simulink model "pattern_separation"  (R2019b)
settings: Solver=FixedStepAuto  StartTime=1  StopTime=simulationtime  FixedStep=stepsize  RelTol=1e-3
values from neighbouring files (symbols this model uses):
  a1 = 0.02    [simulation.m]
  a2 = 0.02    [simulation.m]
  b1 = 0.025    [simulation.m]
  b2 = 0.04    [simulation.m]
  c1 = -65    [simulation.m]
  C1 = normrnd(100,10,[1,nrofgranulecells])    [simulation.m]
  c2 = -65    [simulation.m]
  C2 = normrnd(100,10,[1,nrofinterneurons])    [simulation.m]
  d1 = 6    [simulation.m]
  d2 = 2    [simulation.m]
  inputset = inputsets{no_input}    [simulation.m]
  k1 = 0.25    [simulation.m]
  k2 = 0.25    [simulation.m]
  minimum_saturation_limit_1 = -80    [simulation.m]
  minimum_saturation_limit_2 = -100    [simulation.m]
  noumberofevents = 500    [simulation.m]
  Re = 230    [simulation.m]
  simulationtime = 2000    [simulation.m]
  stepsize = 1    [simulation.m]
  ve1 = -5    [simulation.m]
  ve2 = -80    [simulation.m]
  vr1 = -60    [simulation.m]
  vr2 = -65    [simulation.m]
  vt1 = -55    [simulation.m]
  vt2 = -48    [simulation.m]
undefined symbols (not defined in the file or in its folder): conductancemaxima1, conductancemaxima2, conductancemaxima3, decaytimes1, decaytimes2, decaytimes3, DiscIntNeverNeededParam, Nd, trace
(part 3 of 5)

== system pattern_separation/PV+ interneuron 2/interneuron ==
  postsynaptic current : Inport
  AHP or ADP : Constant  Value=c2  SampleTime=-1
  AP threshold potential : Constant  Value=vt2  SampleTime=-1
  Add : Sum  Inputs=+-
  Add2 : Sum  Inputs=+-
  Add3 : Sum  Inputs=+-
  Constant1 : Constant  Value=d2  SampleTime=-1
  Gain1 : Gain  Gain=b2
  Gain2 : Gain  Gain=k2
  Integrator : Integrator  ExternalReset=rising  InitialCondition=d2
  Integrator1 : Integrator  ExternalReset=rising  InitialCondition=vr2  LimitOutput=on  UpperSaturationLimit=30  LowerSaturationLimit=minimum_saturation_limit_2
  Memory : Memory  InheritSampleTime=on
  Memory1 : Memory  InitialCondition=vr2  InheritSampleTime=on
  Product : Product
  f' : Sum  Inputs=++-
  f'' : Sum  Inputs=+-
  membrne capacitance : Gain  Gain=1/C2(2)
  reset function : MATLAB Function  TreatAsAtomicUnit=on
  resting membrane potential : Constant  Value=vr2  SampleTime=-1
  time constant of relative refractory period : Gain  Gain=a2
  output : Outport
  wires:
  time constant of relative refractory period/1 -> Integrator/1  "u"
  Constant1/1 -> reset function/3(d)
  f''/1 -> time constant of relative refractory period/1
  membrne capacitance/1 -> Integrator1/1  "v"
  resting membrane potential/1 -> Add2/2, Add/2
  AHP or ADP/1 -> reset function/2(c)
  Add2/1 -> Product/1
  reset function/3(r) -> output/1, Integrator1/2, Integrator/2
  Gain1/1 -> f''/1
  Add3/1 -> Product/2
  Memory1/1 -> reset function/1(v)
  reset function/1(v1) -> Add/1, Add2/1, Add3/1
  reset function/2(u1) -> f''/2, f'/3
  Memory/1 -> reset function/4(u)
  Add/1 -> Gain1/1
  Integrator/1 -> Memory/1  "u"
  AP threshold potential/1 -> Add3/2
  Integrator1/1 -> Memory1/1  "v"
  f'/1 -> membrne capacitance/1
  Product/1 -> Gain2/1
  Gain2/1 -> f'/2
  postsynaptic current/1 -> f'/1

== system pattern_separation/PV+ interneuron 2/single exp EPSCs generator (ff synapse) ==
  event time : Inport
  decay time constant : Inport  Port=2
  conductance maximum : Inport  Port=3
  Add1 : Sum  Inputs=+-
  MATLAB Function : MATLAB Function  TreatAsAtomicUnit=on
  Multiply : Gain  Gain=-1
  Product : Product
  Product1 : Product  Inputs=*/
  Product2 : Product
  current reversal potential : Constant  Value=ve1  SampleTime=-1
  resting membrane potential : Constant  Value=vr1  SampleTime=-1
  postsynaptic current : Outport
  wires:
  decay time constant/1 -> Product1/2
  Product/1 -> postsynaptic current/1  "postsynaptic current"
  resting membrane potential/1 -> Add1/1
  current reversal potential/1 -> Add1/2
  conductance maximum/1 -> Product2/2
  Product2/1 -> Product/2  "conductance"
  Add1/1 -> Multiply/1
  Product1/1 -> MATLAB Function/1(inp)
  MATLAB Function/1(exponential) -> Product2/1
  event time/1 -> Product1/1
  Multiply/1 -> Product/1

== system pattern_separation/granule cell 1/granule cell ==
  postsynaptic current : Inport
  AHP or ADP : Constant  Value=c1  SampleTime=-1
  AP threshold potential : Constant  Value=vt1  SampleTime=-1
  Add : Sum  Inputs=+-
  Add2 : Sum  Inputs=+-
  Add3 : Sum  Inputs=+-
  Constant1 : Constant  Value=d1  SampleTime=-1
  Gain1 : Gain  Gain=b1
  Gain2 : Gain  Gain=k1
  Integrator : Integrator  ExternalReset=rising  InitialCondition=d1
  Integrator1 : Integrator  ExternalReset=rising  InitialCondition=vr1  LimitOutput=on  UpperSaturationLimit=30  LowerSaturationLimit=minimum_saturation_limit_1
  Memory : Memory  InheritSampleTime=on
  Memory1 : Memory  InitialCondition=vr1  InheritSampleTime=on
  Product : Product
  f' : Sum  Inputs=++-
  f'' : Sum  Inputs=+-
  membrne capacitance : Gain  Gain=1/C1(1)
  reset function : MATLAB Function  TreatAsAtomicUnit=on
  resting membrane potential : Constant  Value=vr1  SampleTime=-1
  time constant of relative refractory period : Gain  Gain=a1
  v : Outport
  output : Outport  Port=2
  wires:
  time constant of relative refractory period/1 -> Integrator/1  "u"
  Constant1/1 -> reset function/3(d)
  f''/1 -> time constant of relative refractory period/1
  membrne capacitance/1 -> Integrator1/1  "v"
  resting membrane potential/1 -> Add2/2, Add/2
  AHP or ADP/1 -> reset function/2(c)
  Add2/1 -> Product/1
  reset function/3(r) -> output/1, Integrator1/2, Integrator/2
  Gain1/1 -> f''/1
  Add3/1 -> Product/2
  Memory1/1 -> reset function/1(v)
  reset function/1(v1) -> Add/1, Add2/1, Add3/1
  reset function/2(u1) -> f''/2, f'/3
  Memory/1 -> reset function/4(u)
  Add/1 -> Gain1/1
  Integrator/1 -> Memory/1  "u"
  AP threshold potential/1 -> Add3/2
  Integrator1/1 -> v/1, Memory1/1  "v"
  f'/1 -> membrne capacitance/1
  Product/1 -> Gain2/1
  Gain2/1 -> f'/2
  postsynaptic current/1 -> f'/1

== system pattern_separation/granule cell 1/single exp EPSCs generator (recurrent synapse) ==
  event time : Inport
  decay time constant : Inport  Port=2
  conductance maximum : Inport  Port=3
  Add1 : Sum  Inputs=+-
  MATLAB Function : MATLAB Function  TreatAsAtomicUnit=on
  Multiply : Gain  Gain=-1
  Product : Product
  Product1 : Product  Inputs=*/
  Product2 : Product
  current reversal potential : Constant  Value=ve1  SampleTime=-1
  resting membrane potential : Constant  Value=vr1  SampleTime=-1
  postsynaptic current : Outport
  wires:
  decay time constant/1 -> Product1/2
  Product/1 -> postsynaptic current/1  "postsynaptic current"
  resting membrane potential/1 -> Add1/1
  current reversal potential/1 -> Add1/2
  conductance maximum/1 -> Product2/2
  Product2/1 -> Product/2  "conductance"
  Add1/1 -> Multiply/1
  Product1/1 -> MATLAB Function/1(inp)
  MATLAB Function/1(exponential) -> Product2/1
  event time/1 -> Product1/1
  Multiply/1 -> Product/1

== system pattern_separation/granule cell 1/single exp IPSCs generator (ihibitory synapse) ==
  event time : Inport
  decay time constant : Inport  Port=2
  conductance maximum : Inport  Port=3
  Add1 : Sum  Inputs=+-
  MATLAB Function : MATLAB Function  TreatAsAtomicUnit=on
  Multiply : Gain  Gain=-1
  Product : Product
  Product1 : Product  Inputs=*/
  Product2 : Product
  current reversal potential : Constant  Value=ve2  SampleTime=-1
  resting membrane potential : Constant  Value=vr2  SampleTime=-1
  postsynaptic current : Outport
  wires:
  decay time constant/1 -> Product1/2
  Product/1 -> postsynaptic current/1  "postsynaptic current"
  resting membrane potential/1 -> Add1/1
  current reversal potential/1 -> Add1/2
  conductance maximum/1 -> Product2/2
  Product2/1 -> Product/2  "conductance"
  Add1/1 -> Multiply/1
  Product1/1 -> MATLAB Function/1(inp)
  MATLAB Function/1(exponential) -> Product2/1
  event time/1 -> Product1/1
  Multiply/1 -> Product/1

== system pattern_separation/granule cell 10/GC neuron ==
  postsynaptic current : Inport
  AHP or ADP : Constant  Value=c1  SampleTime=-1
  AP threshold potential : Constant  Value=vt1  SampleTime=-1
  Add : Sum  Inputs=+-
  Add2 : Sum  Inputs=+-
  Add3 : Sum  Inputs=+-
  Constant1 : Constant  Value=d1  SampleTime=-1
  Gain1 : Gain  Gain=b1
  Gain2 : Gain  Gain=k1
  Integrator : Integrator  ExternalReset=rising  InitialCondition=d1
  Integrator1 : Integrator  ExternalReset=rising  InitialCondition=vr1  LimitOutput=on  UpperSaturationLimit=30  LowerSaturationLimit=minimum_saturation_limit_1
  Memory : Memory  InheritSampleTime=on
  Memory1 : Memory  InitialCondition=vr1  InheritSampleTime=on
  Product : Product
  f' : Sum  Inputs=++-
  f'' : Sum  Inputs=+-
  membrne capacitance : Gain  Gain=1/C1(10)
  reset function : MATLAB Function  TreatAsAtomicUnit=on
  resting membrane potential : Constant  Value=vr1  SampleTime=-1
  time constant of relative refractory period : Gain  Gain=a1
  v : Outport
  output : Outport  Port=2
  wires:
  time constant of relative refractory period/1 -> Integrator/1  "u"
  Constant1/1 -> reset function/3(d)
  f''/1 -> time constant of relative refractory period/1
  membrne capacitance/1 -> Integrator1/1  "v"
  resting membrane potential/1 -> Add2/2, Add/2
  AHP or ADP/1 -> reset function/2(c)
  Add2/1 -> Product/1
  reset function/3(r) -> Integrator1/2, Integrator/2, output/1
  Gain1/1 -> f''/1
  Add3/1 -> Product/2
  Memory1/1 -> reset function/1(v)
  reset function/1(v1) -> Add/1, Add2/1, Add3/1
  reset function/2(u1) -> f''/2, f'/3
  Memory/1 -> reset function/4(u)
  Add/1 -> Gain1/1
  Integrator/1 -> Memory/1  "u"
  AP threshold potential/1 -> Add3/2
  Integrator1/1 -> v/1, Memory1/1  "v"
  f'/1 -> membrne capacitance/1
  Product/1 -> Gain2/1
  Gain2/1 -> f'/2
  postsynaptic current/1 -> f'/1

== system pattern_separation/granule cell 10/single exp EPSCs generator (recurrent synapse) ==
  event time : Inport
  decay time constant : Inport  Port=2
  conductance maximum : Inport  Port=3
  Add1 : Sum  Inputs=+-
  MATLAB Function : MATLAB Function  TreatAsAtomicUnit=on
  Multiply : Gain  Gain=-1
  Product : Product
  Product1 : Product  Inputs=*/
  Product2 : Product
  current reversal potential : Constant  Value=ve1  SampleTime=-1
  resting membrane potential : Constant  Value=vr1  SampleTime=-1
  postsynaptic current : Outport
  wires:
  decay time constant/1 -> Product1/2
  Product/1 -> postsynaptic current/1  "postsynaptic current"
  resting membrane potential/1 -> Add1/1
  current reversal potential/1 -> Add1/2
  conductance maximum/1 -> Product2/2
  Product2/1 -> Product/2  "conductance"
  Add1/1 -> Multiply/1
  Product1/1 -> MATLAB Function/1(inp)
  MATLAB Function/1(exponential) -> Product2/1
  event time/1 -> Product1/1
  Multiply/1 -> Product/1

== system pattern_separation/granule cell 10/single exp IPSCs generator (ihibitory synapse) ==
  event time : Inport
  decay time constant : Inport  Port=2
  conductance maximum : Inport  Port=3
  Add1 : Sum  Inputs=+-
  MATLAB Function : MATLAB Function  TreatAsAtomicUnit=on
  Multiply : Gain  Gain=-1
  Product : Product
  Product1 : Product  Inputs=*/
  Product2 : Product
  current reversal potential : Constant  Value=ve2  SampleTime=-1
  resting membrane potential : Constant  Value=vr2  SampleTime=-1
  postsynaptic current : Outport
  wires:
  decay time constant/1 -> Product1/2
  Product/1 -> postsynaptic current/1  "postsynaptic current"
  resting membrane potential/1 -> Add1/1
  current reversal potential/1 -> Add1/2
  conductance maximum/1 -> Product2/2
  Product2/1 -> Product/2  "conductance"
  Add1/1 -> Multiply/1
  Product1/1 -> MATLAB Function/1(inp)
  MATLAB Function/1(exponential) -> Product2/1
  event time/1 -> Product1/1
  Multiply/1 -> Product/1

== system pattern_separation/granule cell 11/granule cell ==
  postsynaptic current : Inport
  AHP or ADP : Constant  Value=c1  SampleTime=-1
  AP threshold potential : Constant  Value=vt1  SampleTime=-1
  Add : Sum  Inputs=+-
  Add2 : Sum  Inputs=+-
  Add3 : Sum  Inputs=+-
  Constant1 : Constant  Value=d1  SampleTime=-1
  Gain1 : Gain  Gain=b1
  Gain2 : Gain  Gain=k1
  Integrator : Integrator  ExternalReset=rising  InitialCondition=d1
  Integrator1 : Integrator  ExternalReset=rising  InitialCondition=vr1  LimitOutput=on  UpperSaturationLimit=30  LowerSaturationLimit=minimum_saturation_limit_1
  Memory : Memory  InheritSampleTime=on
  Memory1 : Memory  InitialCondition=vr1  InheritSampleTime=on
  Product : Product
  f' : Sum  Inputs=++-
  f'' : Sum  Inputs=+-
  membrne capacitance : Gain  Gain=1/C1(11)
  reset function : MATLAB Function  TreatAsAtomicUnit=on
  resting membrane potential : Constant  Value=vr1  SampleTime=-1
  time constant of relative refractory period : Gain  Gain=a1
  v : Outport
  output : Outport  Port=2
  wires:
  time constant of relative refractory period/1 -> Integrator/1  "u"
  Constant1/1 -> reset function/3(d)
  f''/1 -> time constant of relative refractory period/1
  membrne capacitance/1 -> Integrator1/1  "v"
  resting membrane potential/1 -> Add2/2, Add/2
  AHP or ADP/1 -> reset function/2(c)
  Add2/1 -> Product/1
  reset function/3(r) -> output/1, Integrator1/2, Integrator/2
  Gain1/1 -> f''/1
  Add3/1 -> Product/2
  Memory1/1 -> reset function/1(v)
  reset function/1(v1) -> Add/1, Add2/1, Add3/1
  reset function/2(u1) -> f''/2, f'/3
  Memory/1 -> reset function/4(u)
  Add/1 -> Gain1/1
  Integrator/1 -> Memory/1  "u"
  AP threshold potential/1 -> Add3/2
  Integrator1/1 -> v/1, Memory1/1  "v"
  f'/1 -> membrne capacitance/1
  Product/1 -> Gain2/1
  Gain2/1 -> f'/2
  postsynaptic current/1 -> f'/1

== system pattern_separation/granule cell 11/single exp EPSCs generator (recurrent synapse) ==
  event time : Inport
  decay time constant : Inport  Port=2
  conductance maximum : Inport  Port=3
  Add1 : Sum  Inputs=+-
  MATLAB Function : MATLAB Function  TreatAsAtomicUnit=on
  Multiply : Gain  Gain=-1
  Product : Product
  Product1 : Product  Inputs=*/
  Product2 : Product
  current reversal potential : Constant  Value=ve1  SampleTime=-1
  resting membrane potential : Constant  Value=vr1  SampleTime=-1
  postsynaptic current : Outport
  wires:
  decay time constant/1 -> Product1/2
  Product/1 -> postsynaptic current/1  "postsynaptic current"
  resting membrane potential/1 -> Add1/1
  current reversal potential/1 -> Add1/2
  conductance maximum/1 -> Product2/2
  Product2/1 -> Product/2  "conductance"
  Add1/1 -> Multiply/1
  Product1/1 -> MATLAB Function/1(inp)
  MATLAB Function/1(exponential) -> Product2/1
  event time/1 -> Product1/1
  Multiply/1 -> Product/1

== system pattern_separation/granule cell 11/single exp IPSCs generator (ihibitory synapse) ==
  event time : Inport
  decay time constant : Inport  Port=2
  conductance maximum : Inport  Port=3
  Add1 : Sum  Inputs=+-
  MATLAB Function : MATLAB Function  TreatAsAtomicUnit=on
  Multiply : Gain  Gain=-1
  Product : Product
  Product1 : Product  Inputs=*/
  Product2 : Product
  current reversal potential : Constant  Value=ve2  SampleTime=-1
  resting membrane potential : Constant  Value=vr2  SampleTime=-1
  postsynaptic current : Outport
  wires:
  decay time constant/1 -> Product1/2
  Product/1 -> postsynaptic current/1  "postsynaptic current"
  resting membrane potential/1 -> Add1/1
  current reversal potential/1 -> Add1/2
  conductance maximum/1 -> Product2/2
  Product2/1 -> Product/2  "conductance"
  Add1/1 -> Multiply/1
  Product1/1 -> MATLAB Function/1(inp)
  MATLAB Function/1(exponential) -> Product2/1
  event time/1 -> Product1/1
  Multiply/1 -> Product/1

== system pattern_separation/granule cell 12/GC neuron ==
  postsynaptic current : Inport
  AHP or ADP : Constant  Value=c1  SampleTime=-1
  AP threshold potential : Constant  Value=vt1  SampleTime=-1
  Add : Sum  Inputs=+-
  Add2 : Sum  Inputs=+-
  Add3 : Sum  Inputs=+-
  Constant1 : Constant  Value=d1  SampleTime=-1
  Gain1 : Gain  Gain=b1
  Gain2 : Gain  Gain=k1
  Integrator : Integrator  ExternalReset=rising  InitialCondition=d1
  Integrator1 : Integrator  ExternalReset=rising  InitialCondition=vr1  LimitOutput=on  UpperSaturationLimit=30  LowerSaturationLimit=minimum_saturation_limit_1
  Memory : Memory  InheritSampleTime=on
  Memory1 : Memory  InitialCondition=vr1  InheritSampleTime=on
  Product : Product
  f' : Sum  Inputs=++-
  f'' : Sum  Inputs=+-
  membrne capacitance : Gain  Gain=1/C1(12)
  reset function : MATLAB Function  TreatAsAtomicUnit=on
  resting membrane potential : Constant  Value=vr1  SampleTime=-1
  time constant of relative refractory period : Gain  Gain=a1
  v : Outport
  output : Outport  Port=2
  wires:
  time constant of relative refractory period/1 -> Integrator/1  "u"
  Constant1/1 -> reset function/3(d)
  f''/1 -> time constant of relative refractory period/1
  membrne capacitance/1 -> Integrator1/1  "v"
  resting membrane potential/1 -> Add2/2, Add/2
  AHP or ADP/1 -> reset function/2(c)
  Add2/1 -> Product/1
  reset function/3(r) -> Integrator1/2, Integrator/2, output/1
  Gain1/1 -> f''/1
  Add3/1 -> Product/2
  Memory1/1 -> reset function/1(v)
  reset function/1(v1) -> Add/1, Add2/1, Add3/1
  reset function/2(u1) -> f''/2, f'/3
  Memory/1 -> reset function/4(u)
  Add/1 -> Gain1/1
  Integrator/1 -> Memory/1  "u"
  AP threshold potential/1 -> Add3/2
  Integrator1/1 -> v/1, Memory1/1  "v"
  f'/1 -> membrne capacitance/1
  Product/1 -> Gain2/1
  Gain2/1 -> f'/2
  postsynaptic current/1 -> f'/1

== system pattern_separation/granule cell 12/single exp EPSCs generator (recurrent synapse) ==
  event time : Inport
  decay time constant : Inport  Port=2
  conductance maximum : Inport  Port=3
  Add1 : Sum  Inputs=+-
  MATLAB Function : MATLAB Function  TreatAsAtomicUnit=on
  Multiply : Gain  Gain=-1
  Product : Product
  Product1 : Product  Inputs=*/
  Product2 : Product
  current reversal potential : Constant  Value=ve1  SampleTime=-1
  resting membrane potential : Constant  Value=vr1  SampleTime=-1
  postsynaptic current : Outport
  wires:
  decay time constant/1 -> Product1/2
  Product/1 -> postsynaptic current/1  "postsynaptic current"
  resting membrane potential/1 -> Add1/1
  current reversal potential/1 -> Add1/2
  conductance maximum/1 -> Product2/2
  Product2/1 -> Product/2  "conductance"
  Add1/1 -> Multiply/1
  Product1/1 -> MATLAB Function/1(inp)
  MATLAB Function/1(exponential) -> Product2/1
  event time/1 -> Product1/1
  Multiply/1 -> Product/1

== system pattern_separation/granule cell 12/single exp IPSCs generator (ihibitory synapse) ==
  event time : Inport
  decay time constant : Inport  Port=2
  conductance maximum : Inport  Port=3
  Add1 : Sum  Inputs=+-
  MATLAB Function : MATLAB Function  TreatAsAtomicUnit=on
  Multiply : Gain  Gain=-1
  Product : Product
  Product1 : Product  Inputs=*/
  Product2 : Product
  current reversal potential : Constant  Value=ve2  SampleTime=-1
  resting membrane potential : Constant  Value=vr2  SampleTime=-1
  postsynaptic current : Outport
  wires:
  decay time constant/1 -> Product1/2
  Product/1 -> postsynaptic current/1  "postsynaptic current"
  resting membrane potential/1 -> Add1/1
  current reversal potential/1 -> Add1/2
  conductance maximum/1 -> Product2/2
  Product2/1 -> Product/2  "conductance"
  Add1/1 -> Multiply/1
  Product1/1 -> MATLAB Function/1(inp)
  MATLAB Function/1(exponential) -> Product2/1
  event time/1 -> Product1/1
  Multiply/1 -> Product/1

== system pattern_separation/granule cell 13/granule cell ==
  postsynaptic current : Inport
  AHP or ADP : Constant  Value=c1  SampleTime=-1
  AP threshold potential : Constant  Value=vt1  SampleTime=-1
  Add : Sum  Inputs=+-
  Add2 : Sum  Inputs=+-
  Add3 : Sum  Inputs=+-
  Constant1 : Constant  Value=d1  SampleTime=-1
  Gain1 : Gain  Gain=b1
  Gain2 : Gain  Gain=k1
  Integrator : Integrator  ExternalReset=rising  InitialCondition=d1
  Integrator1 : Integrator  ExternalReset=rising  InitialCondition=vr1  LimitOutput=on  UpperSaturationLimit=30  LowerSaturationLimit=minimum_saturation_limit_1
  Memory : Memory  InheritSampleTime=on
  Memory1 : Memory  InitialCondition=vr1  InheritSampleTime=on
  Product : Product
  f' : Sum  Inputs=++-
  f'' : Sum  Inputs=+-
  membrne capacitance : Gain  Gain=1/C1(13)
  reset function : MATLAB Function  TreatAsAtomicUnit=on
  resting membrane potential : Constant  Value=vr1  SampleTime=-1
  time constant of relative refractory period : Gain  Gain=a1
  v : Outport
  output : Outport  Port=2
  wires:
  time constant of relative refractory period/1 -> Integrator/1  "u"
  Constant1/1 -> reset function/3(d)
  f''/1 -> time constant of relative refractory period/1
  membrne capacitance/1 -> Integrator1/1  "v"
  resting membrane potential/1 -> Add2/2, Add/2
  AHP or ADP/1 -> reset function/2(c)
  Add2/1 -> Product/1
  reset function/3(r) -> output/1, Integrator1/2, Integrator/2
  Gain1/1 -> f''/1
  Add3/1 -> Product/2
  Memory1/1 -> reset function/1(v)
  reset function/1(v1) -> Add/1, Add2/1, Add3/1
  reset function/2(u1) -> f''/2, f'/3
  Memory/1 -> reset function/4(u)
  Add/1 -> Gain1/1
  Integrator/1 -> Memory/1  "u"
  AP threshold potential/1 -> Add3/2
  Integrator1/1 -> v/1, Memory1/1  "v"
  f'/1 -> membrne capacitance/1
  Product/1 -> Gain2/1
  Gain2/1 -> f'/2
  postsynaptic current/1 -> f'/1

== system pattern_separation/granule cell 13/single exp EPSCs generator (recurrent synapse) ==
  event time : Inport
  decay time constant : Inport  Port=2
  conductance maximum : Inport  Port=3
  Add1 : Sum  Inputs=+-
  MATLAB Function : MATLAB Function  TreatAsAtomicUnit=on
  Multiply : Gain  Gain=-1
  Product : Product
  Product1 : Product  Inputs=*/
  Product2 : Product
  current reversal potential : Constant  Value=ve1  SampleTime=-1
  resting membrane potential : Constant  Value=vr1  SampleTime=-1
  postsynaptic current : Outport
  wires:
  decay time constant/1 -> Product1/2
  Product/1 -> postsynaptic current/1  "postsynaptic current"
  resting membrane potential/1 -> Add1/1
  current reversal potential/1 -> Add1/2
  conductance maximum/1 -> Product2/2
  Product2/1 -> Product/2  "conductance"
  Add1/1 -> Multiply/1
  Product1/1 -> MATLAB Function/1(inp)
  MATLAB Function/1(exponential) -> Product2/1
  event time/1 -> Product1/1
  Multiply/1 -> Product/1

== system pattern_separation/granule cell 13/single exp IPSCs generator (ihibitory synapse) ==
  event time : Inport
  decay time constant : Inport  Port=2
  conductance maximum : Inport  Port=3
  Add1 : Sum  Inputs=+-
  MATLAB Function : MATLAB Function  TreatAsAtomicUnit=on
  Multiply : Gain  Gain=-1
  Product : Product
  Product1 : Product  Inputs=*/
  Product2 : Product
  current reversal potential : Constant  Value=ve2  SampleTime=-1
  resting membrane potential : Constant  Value=vr2  SampleTime=-1
  postsynaptic current : Outport
  wires:
  decay time constant/1 -> Product1/2
  Product/1 -> postsynaptic current/1  "postsynaptic current"
  resting membrane potential/1 -> Add1/1
  current reversal potential/1 -> Add1/2
  conductance maximum/1 -> Product2/2
  Product2/1 -> Product/2  "conductance"
  Add1/1 -> Multiply/1
  Product1/1 -> MATLAB Function/1(inp)
  MATLAB Function/1(exponential) -> Product2/1
  event time/1 -> Product1/1
  Multiply/1 -> Product/1

== system pattern_separation/granule cell 14/GC neuron ==
  postsynaptic current : Inport
  AHP or ADP : Constant  Value=c1  SampleTime=-1
  AP threshold potential : Constant  Value=vt1  SampleTime=-1
  Add : Sum  Inputs=+-
  Add2 : Sum  Inputs=+-
  Add3 : Sum  Inputs=+-
  Constant1 : Constant  Value=d1  SampleTime=-1
  Gain1 : Gain  Gain=b1
  Gain2 : Gain  Gain=k1
  Integrator : Integrator  ExternalReset=rising  InitialCondition=d1
  Integrator1 : Integrator  ExternalReset=rising  InitialCondition=vr1  LimitOutput=on  UpperSaturationLimit=30  LowerSaturationLimit=minimum_saturation_limit_1
  Memory : Memory  InheritSampleTime=on
  Memory1 : Memory  InitialCondition=vr1  InheritSampleTime=on
  Product : Product
  f' : Sum  Inputs=++-
  f'' : Sum  Inputs=+-
  membrne capacitance : Gain  Gain=1/C1(14)
  reset function : MATLAB Function  TreatAsAtomicUnit=on
  resting membrane potential : Constant  Value=vr1  SampleTime=-1
  time constant of relative refractory period : Gain  Gain=a1
  v : Outport
  output : Outport  Port=2
  wires:
  time constant of relative refractory period/1 -> Integrator/1  "u"
  Constant1/1 -> reset function/3(d)
  f''/1 -> time constant of relative refractory period/1
  membrne capacitance/1 -> Integrator1/1  "v"
  resting membrane potential/1 -> Add2/2, Add/2
  AHP or ADP/1 -> reset function/2(c)
  Add2/1 -> Product/1
  reset function/3(r) -> Integrator1/2, Integrator/2, output/1
  Gain1/1 -> f''/1
  Add3/1 -> Product/2
  Memory1/1 -> reset function/1(v)
  reset function/1(v1) -> Add/1, Add2/1, Add3/1
  reset function/2(u1) -> f''/2, f'/3
  Memory/1 -> reset function/4(u)
  Add/1 -> Gain1/1
  Integrator/1 -> Memory/1  "u"
  AP threshold potential/1 -> Add3/2
  Integrator1/1 -> v/1, Memory1/1  "v"
  f'/1 -> membrne capacitance/1
  Product/1 -> Gain2/1
  Gain2/1 -> f'/2
  postsynaptic current/1 -> f'/1

== system pattern_separation/granule cell 14/single exp EPSCs generator (recurrent synapse) ==
  event time : Inport
  decay time constant : Inport  Port=2
  conductance maximum : Inport  Port=3
  Add1 : Sum  Inputs=+-
  MATLAB Function : MATLAB Function  TreatAsAtomicUnit=on
  Multiply : Gain  Gain=-1
  Product : Product
  Product1 : Product  Inputs=*/
  Product2 : Product
  current reversal potential : Constant  Value=ve1  SampleTime=-1
  resting membrane potential : Constant  Value=vr1  SampleTime=-1
  postsynaptic current : Outport
  wires:
  decay time constant/1 -> Product1/2
  Product/1 -> postsynaptic current/1  "postsynaptic current"
  resting membrane potential/1 -> Add1/1
  current reversal potential/1 -> Add1/2
  conductance maximum/1 -> Product2/2
  Product2/1 -> Product/2  "conductance"
  Add1/1 -> Multiply/1
  Product1/1 -> MATLAB Function/1(inp)
  MATLAB Function/1(exponential) -> Product2/1
  event time/1 -> Product1/1
  Multiply/1 -> Product/1

== system pattern_separation/granule cell 14/single exp IPSCs generator (ihibitory synapse) ==
  event time : Inport
  decay time constant : Inport  Port=2
  conductance maximum : Inport  Port=3
  Add1 : Sum  Inputs=+-
  MATLAB Function : MATLAB Function  TreatAsAtomicUnit=on
  Multiply : Gain  Gain=-1
  Product : Product
  Product1 : Product  Inputs=*/
  Product2 : Product
  current reversal potential : Constant  Value=ve2  SampleTime=-1
  resting membrane potential : Constant  Value=vr2  SampleTime=-1
  postsynaptic current : Outport
  wires:
  decay time constant/1 -> Product1/2
  Product/1 -> postsynaptic current/1  "postsynaptic current"
  resting membrane potential/1 -> Add1/1
  current reversal potential/1 -> Add1/2
  conductance maximum/1 -> Product2/2
  Product2/1 -> Product/2  "conductance"
  Add1/1 -> Multiply/1
  Product1/1 -> MATLAB Function/1(inp)
  MATLAB Function/1(exponential) -> Product2/1
  event time/1 -> Product1/1
  Multiply/1 -> Product/1

== system pattern_separation/granule cell 15/granule cell ==
  postsynaptic current : Inport
  AHP or ADP : Constant  Value=c1  SampleTime=-1
  AP threshold potential : Constant  Value=vt1  SampleTime=-1
  Add : Sum  Inputs=+-
  Add2 : Sum  Inputs=+-
  Add3 : Sum  Inputs=+-
  Constant1 : Constant  Value=d1  SampleTime=-1
  Gain1 : Gain  Gain=b1
  Gain2 : Gain  Gain=k1
  Integrator : Integrator  ExternalReset=rising  InitialCondition=d1
  Integrator1 : Integrator  ExternalReset=rising  InitialCondition=vr1  LimitOutput=on  UpperSaturationLimit=30  LowerSaturationLimit=minimum_saturation_limit_1
  Memory : Memory  InheritSampleTime=on
  Memory1 : Memory  InitialCondition=vr1  InheritSampleTime=on
  Product : Product
  f' : Sum  Inputs=++-
  f'' : Sum  Inputs=+-
  membrne capacitance : Gain  Gain=1/C1(15)
  reset function : MATLAB Function  TreatAsAtomicUnit=on
  resting membrane potential : Constant  Value=vr1  SampleTime=-1
  time constant of relative refractory period : Gain  Gain=a1
  v : Outport
  output : Outport  Port=2
  wires:
  time constant of relative refractory period/1 -> Integrator/1  "u"
  Constant1/1 -> reset function/3(d)
  f''/1 -> time constant of relative refractory period/1
  membrne capacitance/1 -> Integrator1/1  "v"
  resting membrane potential/1 -> Add2/2, Add/2
  AHP or ADP/1 -> reset function/2(c)
  Add2/1 -> Product/1
  reset function/3(r) -> output/1, Integrator1/2, Integrator/2
  Gain1/1 -> f''/1
  Add3/1 -> Product/2
  Memory1/1 -> reset function/1(v)
  reset function/1(v1) -> Add/1, Add2/1, Add3/1
  reset function/2(u1) -> f''/2, f'/3
  Memory/1 -> reset function/4(u)
  Add/1 -> Gain1/1
  Integrator/1 -> Memory/1  "u"
  AP threshold potential/1 -> Add3/2
  Integrator1/1 -> v/1, Memory1/1  "v"
  f'/1 -> membrne capacitance/1
  Product/1 -> Gain2/1
  Gain2/1 -> f'/2
  postsynaptic current/1 -> f'/1

== system pattern_separation/granule cell 15/single exp EPSCs generator (recurrent synapse) ==
  event time : Inport
  decay time constant : Inport  Port=2
  conductance maximum : Inport  Port=3
  Add1 : Sum  Inputs=+-
  MATLAB Function : MATLAB Function  TreatAsAtomicUnit=on
  Multiply : Gain  Gain=-1
  Product : Product
  Product1 : Product  Inputs=*/
  Product2 : Product
  current reversal potential : Constant  Value=ve1  SampleTime=-1
  resting membrane potential : Constant  Value=vr1  SampleTime=-1
  postsynaptic current : Outport
  wires:
  decay time constant/1 -> Product1/2
  Product/1 -> postsynaptic current/1  "postsynaptic current"
  resting membrane potential/1 -> Add1/1
  current reversal potential/1 -> Add1/2
  conductance maximum/1 -> Product2/2
  Product2/1 -> Product/2  "conductance"
  Add1/1 -> Multiply/1
  Product1/1 -> MATLAB Function/1(inp)
  MATLAB Function/1(exponential) -> Product2/1
  event time/1 -> Product1/1
  Multiply/1 -> Product/1

== system pattern_separation/granule cell 15/single exp IPSCs generator (ihibitory synapse) ==
  event time : Inport
  decay time constant : Inport  Port=2
  conductance maximum : Inport  Port=3
  Add1 : Sum  Inputs=+-
  MATLAB Function : MATLAB Function  TreatAsAtomicUnit=on
  Multiply : Gain  Gain=-1
  Product : Product
  Product1 : Product  Inputs=*/
  Product2 : Product
  current reversal potential : Constant  Value=ve2  SampleTime=-1
  resting membrane potential : Constant  Value=vr2  SampleTime=-1
  postsynaptic current : Outport
  wires:
  decay time constant/1 -> Product1/2
  Product/1 -> postsynaptic current/1  "postsynaptic current"
  resting membrane potential/1 -> Add1/1
  current reversal potential/1 -> Add1/2
  conductance maximum/1 -> Product2/2
  Product2/1 -> Product/2  "conductance"
  Add1/1 -> Multiply/1
  Product1/1 -> MATLAB Function/1(inp)
  MATLAB Function/1(exponential) -> Product2/1
  event time/1 -> Product1/1
  Multiply/1 -> Product/1

== system pattern_separation/granule cell 16/GC neuron ==
  postsynaptic current : Inport
  AHP or ADP : Constant  Value=c1  SampleTime=-1
  AP threshold potential : Constant  Value=vt1  SampleTime=-1
  Add : Sum  Inputs=+-
  Add2 : Sum  Inputs=+-
  Add3 : Sum  Inputs=+-
  Constant1 : Constant  Value=d1  SampleTime=-1
  Gain1 : Gain  Gain=b1
  Gain2 : Gain  Gain=k1
  Integrator : Integrator  ExternalReset=rising  InitialCondition=d1
  Integrator1 : Integrator  ExternalReset=rising  InitialCondition=vr1  LimitOutput=on  UpperSaturationLimit=30  LowerSaturationLimit=minimum_saturation_limit_1
  Memory : Memory  InheritSampleTime=on
  Memory1 : Memory  InitialCondition=vr1  InheritSampleTime=on
  Product : Product
  f' : Sum  Inputs=++-
  f'' : Sum  Inputs=+-
  membrne capacitance : Gain  Gain=1/C1(16)
  reset function : MATLAB Function  TreatAsAtomicUnit=on
  resting membrane potential : Constant  Value=vr1  SampleTime=-1
  time constant of relative refractory period : Gain  Gain=a1
  v : Outport
  output : Outport  Port=2
  wires:
  time constant of relative refractory period/1 -> Integrator/1  "u"
  Constant1/1 -> reset function/3(d)
  f''/1 -> time constant of relative refractory period/1
  membrne capacitance/1 -> Integrator1/1  "v"
  resting membrane potential/1 -> Add2/2, Add/2
  AHP or ADP/1 -> reset function/2(c)
  Add2/1 -> Product/1
  reset function/3(r) -> Integrator1/2, Integrator/2, output/1
  Gain1/1 -> f''/1
  Add3/1 -> Product/2
  Memory1/1 -> reset function/1(v)
  reset function/1(v1) -> Add/1, Add2/1, Add3/1
  reset function/2(u1) -> f''/2, f'/3
  Memory/1 -> reset function/4(u)
  Add/1 -> Gain1/1
  Integrator/1 -> Memory/1  "u"
  AP threshold potential/1 -> Add3/2
  Integrator1/1 -> v/1, Memory1/1  "v"
  f'/1 -> membrne capacitance/1
  Product/1 -> Gain2/1
  Gain2/1 -> f'/2
  postsynaptic current/1 -> f'/1

== system pattern_separation/granule cell 16/single exp EPSCs generator (recurrent synapse) ==
  event time : Inport
  decay time constant : Inport  Port=2
  conductance maximum : Inport  Port=3
  Add1 : Sum  Inputs=+-
  MATLAB Function : MATLAB Function  TreatAsAtomicUnit=on
  Multiply : Gain  Gain=-1
  Product : Product
  Product1 : Product  Inputs=*/
  Product2 : Product
  current reversal potential : Constant  Value=ve1  SampleTime=-1
  resting membrane potential : Constant  Value=vr1  SampleTime=-1
  postsynaptic current : Outport
  wires:
  decay time constant/1 -> Product1/2
  Product/1 -> postsynaptic current/1  "postsynaptic current"
  resting membrane potential/1 -> Add1/1
  current reversal potential/1 -> Add1/2
  conductance maximum/1 -> Product2/2
  Product2/1 -> Product/2  "conductance"
  Add1/1 -> Multiply/1
  Product1/1 -> MATLAB Function/1(inp)
  MATLAB Function/1(exponential) -> Product2/1
  event time/1 -> Product1/1
  Multiply/1 -> Product/1

== system pattern_separation/granule cell 16/single exp IPSCs generator (ihibitory synapse) ==
  event time : Inport
  decay time constant : Inport  Port=2
  conductance maximum : Inport  Port=3
  Add1 : Sum  Inputs=+-
  MATLAB Function : MATLAB Function  TreatAsAtomicUnit=on
  Multiply : Gain  Gain=-1
  Product : Product
  Product1 : Product  Inputs=*/
  Product2 : Product
  current reversal potential : Constant  Value=ve2  SampleTime=-1
  resting membrane potential : Constant  Value=vr2  SampleTime=-1
  postsynaptic current : Outport
  wires:
  decay time constant/1 -> Product1/2
  Product/1 -> postsynaptic current/1  "postsynaptic current"
  resting membrane potential/1 -> Add1/1
  current reversal potential/1 -> Add1/2
  conductance maximum/1 -> Product2/2
  Product2/1 -> Product/2  "conductance"
  Add1/1 -> Multiply/1
  Product1/1 -> MATLAB Function/1(inp)
  MATLAB Function/1(exponential) -> Product2/1
  event time/1 -> Product1/1
  Multiply/1 -> Product/1

== system pattern_separation/granule cell 17/granule cell ==
  postsynaptic current : Inport
  AHP or ADP : Constant  Value=c1  SampleTime=-1
  AP threshold potential : Constant  Value=vt1  SampleTime=-1
  Add : Sum  Inputs=+-
  Add2 : Sum  Inputs=+-
  Add3 : Sum  Inputs=+-
  Constant1 : Constant  Value=d1  SampleTime=-1
  Gain1 : Gain  Gain=b1
  Gain2 : Gain  Gain=k1
  Integrator : Integrator  ExternalReset=rising  InitialCondition=d1
  Integrator1 : Integrator  ExternalReset=rising  InitialCondition=vr1  LimitOutput=on  UpperSaturationLimit=30  LowerSaturationLimit=minimum_saturation_limit_1
  Memory : Memory  InheritSampleTime=on
  Memory1 : Memory  InitialCondition=vr1  InheritSampleTime=on
  Product : Product
  f' : Sum  Inputs=++-
  f'' : Sum  Inputs=+-
  membrne capacitance : Gain  Gain=1/C1(17)
  reset function : MATLAB Function  TreatAsAtomicUnit=on
  resting membrane potential : Constant  Value=vr1  SampleTime=-1
  time constant of relative refractory period : Gain  Gain=a1
  v : Outport
  output : Outport  Port=2
  wires:
  time constant of relative refractory period/1 -> Integrator/1  "u"
  Constant1/1 -> reset function/3(d)
  f''/1 -> time constant of relative refractory period/1
  membrne capacitance/1 -> Integrator1/1  "v"
  resting membrane potential/1 -> Add2/2, Add/2
  AHP or ADP/1 -> reset function/2(c)
  Add2/1 -> Product/1
  reset function/3(r) -> output/1, Integrator1/2, Integrator/2
  Gain1/1 -> f''/1
  Add3/1 -> Product/2
  Memory1/1 -> reset function/1(v)
  reset function/1(v1) -> Add/1, Add2/1, Add3/1
  reset function/2(u1) -> f''/2, f'/3
  Memory/1 -> reset function/4(u)
  Add/1 -> Gain1/1
  Integrator/1 -> Memory/1  "u"
  AP threshold potential/1 -> Add3/2
  Integrator1/1 -> v/1, Memory1/1  "v"
  f'/1 -> membrne capacitance/1
  Product/1 -> Gain2/1
  Gain2/1 -> f'/2
  postsynaptic current/1 -> f'/1

== system pattern_separation/granule cell 17/single exp EPSCs generator (recurrent synapse) ==
  event time : Inport
  decay time constant : Inport  Port=2
  conductance maximum : Inport  Port=3
  Add1 : Sum  Inputs=+-
  MATLAB Function : MATLAB Function  TreatAsAtomicUnit=on
  Multiply : Gain  Gain=-1
  Product : Product
  Product1 : Product  Inputs=*/
  Product2 : Product
  current reversal potential : Constant  Value=ve1  SampleTime=-1
  resting membrane potential : Constant  Value=vr1  SampleTime=-1
  postsynaptic current : Outport
  wires:
  decay time constant/1 -> Product1/2
  Product/1 -> postsynaptic current/1  "postsynaptic current"
  resting membrane potential/1 -> Add1/1
  current reversal potential/1 -> Add1/2
  conductance maximum/1 -> Product2/2
  Product2/1 -> Product/2  "conductance"
  Add1/1 -> Multiply/1
  Product1/1 -> MATLAB Function/1(inp)
  MATLAB Function/1(exponential) -> Product2/1
  event time/1 -> Product1/1
  Multiply/1 -> Product/1

== system pattern_separation/granule cell 17/single exp IPSCs generator (ihibitory synapse) ==
  event time : Inport
  decay time constant : Inport  Port=2
  conductance maximum : Inport  Port=3
  Add1 : Sum  Inputs=+-
  MATLAB Function : MATLAB Function  TreatAsAtomicUnit=on
  Multiply : Gain  Gain=-1
  Product : Product
  Product1 : Product  Inputs=*/
  Product2 : Product
  current reversal potential : Constant  Value=ve2  SampleTime=-1
  resting membrane potential : Constant  Value=vr2  SampleTime=-1
  postsynaptic current : Outport
  wires:
  decay time constant/1 -> Product1/2
  Product/1 -> postsynaptic current/1  "postsynaptic current"
  resting membrane potential/1 -> Add1/1
  current reversal potential/1 -> Add1/2
  conductance maximum/1 -> Product2/2
  Product2/1 -> Product/2  "conductance"
  Add1/1 -> Multiply/1
  Product1/1 -> MATLAB Function/1(inp)
  MATLAB Function/1(exponential) -> Product2/1
  event time/1 -> Product1/1
  Multiply/1 -> Product/1

== system pattern_separation/granule cell 18/GC neuron ==
  postsynaptic current : Inport
  AHP or ADP : Constant  Value=c1  SampleTime=-1
  AP threshold potential : Constant  Value=vt1  SampleTime=-1
  Add : Sum  Inputs=+-
  Add2 : Sum  Inputs=+-
  Add3 : Sum  Inputs=+-
  Constant1 : Constant  Value=d1  SampleTime=-1
  Gain1 : Gain  Gain=b1
  Gain2 : Gain  Gain=k1
  Integrator : Integrator  ExternalReset=rising  InitialCondition=d1
  Integrator1 : Integrator  ExternalReset=rising  InitialCondition=vr1  LimitOutput=on  UpperSaturationLimit=30  LowerSaturationLimit=minimum_saturation_limit_1
  Memory : Memory  InheritSampleTime=on
  Memory1 : Memory  InitialCondition=vr1  InheritSampleTime=on
  Product : Product
  f' : Sum  Inputs=++-
  f'' : Sum  Inputs=+-
  membrne capacitance : Gain  Gain=1/C1(18)
  reset function : MATLAB Function  TreatAsAtomicUnit=on
  resting membrane potential : Constant  Value=vr1  SampleTime=-1
  time constant of relative refractory period : Gain  Gain=a1
  v : Outport
  output : Outport  Port=2
  wires:
  time constant of relative refractory period/1 -> Integrator/1  "u"
  Constant1/1 -> reset function/3(d)
  f''/1 -> time constant of relative refractory period/1
  membrne capacitance/1 -> Integrator1/1  "v"
  resting membrane potential/1 -> Add2/2, Add/2
  AHP or ADP/1 -> reset function/2(c)
  Add2/1 -> Product/1
  reset function/3(r) -> Integrator1/2, Integrator/2, output/1
  Gain1/1 -> f''/1
  Add3/1 -> Product/2
  Memory1/1 -> reset function/1(v)
  reset function/1(v1) -> Add/1, Add2/1, Add3/1
  reset function/2(u1) -> f''/2, f'/3
  Memory/1 -> reset function/4(u)
  Add/1 -> Gain1/1
  Integrator/1 -> Memory/1  "u"
  AP threshold potential/1 -> Add3/2
  Integrator1/1 -> v/1, Memory1/1  "v"
  f'/1 -> membrne capacitance/1
  Product/1 -> Gain2/1
  Gain2/1 -> f'/2
  postsynaptic current/1 -> f'/1

== system pattern_separation/granule cell 18/single exp EPSCs generator (recurrent synapse) ==
  event time : Inport
  decay time constant : Inport  Port=2
  conductance maximum : Inport  Port=3
  Add1 : Sum  Inputs=+-
  MATLAB Function : MATLAB Function  TreatAsAtomicUnit=on
  Multiply : Gain  Gain=-1
  Product : Product
  Product1 : Product  Inputs=*/
  Product2 : Product
  current reversal potential : Constant  Value=ve1  SampleTime=-1
  resting membrane potential : Constant  Value=vr1  SampleTime=-1
  postsynaptic current : Outport
  wires:
  decay time constant/1 -> Product1/2
  Product/1 -> postsynaptic current/1  "postsynaptic current"
  resting membrane potential/1 -> Add1/1
  current reversal potential/1 -> Add1/2
  conductance maximum/1 -> Product2/2
  Product2/1 -> Product/2  "conductance"
  Add1/1 -> Multiply/1
  Product1/1 -> MATLAB Function/1(inp)
  MATLAB Function/1(exponential) -> Product2/1
  event time/1 -> Product1/1
  Multiply/1 -> Product/1

== system pattern_separation/granule cell 18/single exp IPSCs generator (ihibitory synapse) ==
  event time : Inport
  decay time constant : Inport  Port=2
  conductance maximum : Inport  Port=3
  Add1 : Sum  Inputs=+-
  MATLAB Function : MATLAB Function  TreatAsAtomicUnit=on
  Multiply : Gain  Gain=-1
  Product : Product
  Product1 : Product  Inputs=*/
  Product2 : Product
  current reversal potential : Constant  Value=ve2  SampleTime=-1
  resting membrane potential : Constant  Value=vr2  SampleTime=-1
  postsynaptic current : Outport
  wires:
  decay time constant/1 -> Product1/2
  Product/1 -> postsynaptic current/1  "postsynaptic current"
  resting membrane potential/1 -> Add1/1
  current reversal potential/1 -> Add1/2
  conductance maximum/1 -> Product2/2
  Product2/1 -> Product/2  "conductance"
  Add1/1 -> Multiply/1
  Product1/1 -> MATLAB Function/1(inp)
  MATLAB Function/1(exponential) -> Product2/1
  event time/1 -> Product1/1
  Multiply/1 -> Product/1

== system pattern_separation/granule cell 19/granule cell ==
  postsynaptic current : Inport
  AHP or ADP : Constant  Value=c1  SampleTime=-1
  AP threshold potential : Constant  Value=vt1  SampleTime=-1
  Add : Sum  Inputs=+-
  Add2 : Sum  Inputs=+-
  Add3 : Sum  Inputs=+-
  Constant1 : Constant  Value=d1  SampleTime=-1
  Gain1 : Gain  Gain=b1
  Gain2 : Gain  Gain=k1
  Integrator : Integrator  ExternalReset=rising  InitialCondition=d1
  Integrator1 : Integrator  ExternalReset=rising  InitialCondition=vr1  LimitOutput=on  UpperSaturationLimit=30  LowerSaturationLimit=minimum_saturation_limit_1
  Memory : Memory  InheritSampleTime=on
  Memory1 : Memory  InitialCondition=vr1  InheritSampleTime=on
  Product : Product
  f' : Sum  Inputs=++-
  f'' : Sum  Inputs=+-
  membrne capacitance : Gain  Gain=1/C1(19)
  reset function : MATLAB Function  TreatAsAtomicUnit=on
  resting membrane potential : Constant  Value=vr1  SampleTime=-1
  time constant of relative refractory period : Gain  Gain=a1
  v : Outport
  output : Outport  Port=2
  wires:
  time constant of relative refractory period/1 -> Integrator/1  "u"
  Constant1/1 -> reset function/3(d)
  f''/1 -> time constant of relative refractory period/1
  membrne capacitance/1 -> Integrator1/1  "v"
  resting membrane potential/1 -> Add2/2, Add/2
  AHP or ADP/1 -> reset function/2(c)
  Add2/1 -> Product/1
  reset function/3(r) -> output/1, Integrator1/2, Integrator/2
  Gain1/1 -> f''/1
  Add3/1 -> Product/2
  Memory1/1 -> reset function/1(v)
  reset function/1(v1) -> Add/1, Add2/1, Add3/1
  reset function/2(u1) -> f''/2, f'/3
  Memory/1 -> reset function/4(u)
  Add/1 -> Gain1/1
  Integrator/1 -> Memory/1  "u"
  AP threshold potential/1 -> Add3/2
  Integrator1/1 -> v/1, Memory1/1  "v"
  f'/1 -> membrne capacitance/1
  Product/1 -> Gain2/1
  Gain2/1 -> f'/2
  postsynaptic current/1 -> f'/1

== system pattern_separation/granule cell 19/single exp EPSCs generator (recurrent synapse) ==
  event time : Inport
  decay time constant : Inport  Port=2
  conductance maximum : Inport  Port=3
  Add1 : Sum  Inputs=+-
  MATLAB Function : MATLAB Function  TreatAsAtomicUnit=on
  Multiply : Gain  Gain=-1
  Product : Product
  Product1 : Product  Inputs=*/
  Product2 : Product
  current reversal potential : Constant  Value=ve1  SampleTime=-1
  resting membrane potential : Constant  Value=vr1  SampleTime=-1
  postsynaptic current : Outport
  wires:
  decay time constant/1 -> Product1/2
  Product/1 -> postsynaptic current/1  "postsynaptic current"
  resting membrane potential/1 -> Add1/1
  current reversal potential/1 -> Add1/2
  conductance maximum/1 -> Product2/2
  Product2/1 -> Product/2  "conductance"
  Add1/1 -> Multiply/1
  Product1/1 -> MATLAB Function/1(inp)
  MATLAB Function/1(exponential) -> Product2/1
  event time/1 -> Product1/1
  Multiply/1 -> Product/1

== system pattern_separation/granule cell 19/single exp IPSCs generator (ihibitory synapse) ==
  event time : Inport
  decay time constant : Inport  Port=2
  conductance maximum : Inport  Port=3
  Add1 : Sum  Inputs=+-
  MATLAB Function : MATLAB Function  TreatAsAtomicUnit=on
  Multiply : Gain  Gain=-1
  Product : Product
  Product1 : Product  Inputs=*/
  Product2 : Product
  current reversal potential : Constant  Value=ve2  SampleTime=-1
  resting membrane potential : Constant  Value=vr2  SampleTime=-1
  postsynaptic current : Outport
  wires:
  decay time constant/1 -> Product1/2
  Product/1 -> postsynaptic current/1  "postsynaptic current"
  resting membrane potential/1 -> Add1/1
  current reversal potential/1 -> Add1/2
  conductance maximum/1 -> Product2/2
  Product2/1 -> Product/2  "conductance"
  Add1/1 -> Multiply/1
  Product1/1 -> MATLAB Function/1(inp)
  MATLAB Function/1(exponential) -> Product2/1
  event time/1 -> Product1/1
  Multiply/1 -> Product/1

== system pattern_separation/granule cell 2/GC neuron ==
  postsynaptic current : Inport
  AHP or ADP : Constant  Value=c1  SampleTime=-1
  AP threshold potential : Constant  Value=vt1  SampleTime=-1
  Add : Sum  Inputs=+-
  Add2 : Sum  Inputs=+-
  Add3 : Sum  Inputs=+-
  Constant1 : Constant  Value=d1  SampleTime=-1
  Gain1 : Gain  Gain=b1
  Gain2 : Gain  Gain=k1
  Integrator : Integrator  ExternalReset=rising  InitialCondition=d1
  Integrator1 : Integrator  ExternalReset=rising  InitialCondition=vr1  LimitOutput=on  UpperSaturationLimit=30  LowerSaturationLimit=minimum_saturation_limit_1
  Memory : Memory  InheritSampleTime=on
  Memory1 : Memory  InitialCondition=vr1  InheritSampleTime=on
  Product : Product
  f' : Sum  Inputs=++-
  f'' : Sum  Inputs=+-
  membrne capacitance : Gain  Gain=1/C1(2)
  reset function : MATLAB Function  TreatAsAtomicUnit=on
  resting membrane potential : Constant  Value=vr1  SampleTime=-1
  time constant of relative refractory period : Gain  Gain=a1
  v : Outport
  output : Outport  Port=2
  wires:
  time constant of relative refractory period/1 -> Integrator/1  "u"
  Constant1/1 -> reset function/3(d)
  f''/1 -> time constant of relative refractory period/1
  membrne capacitance/1 -> Integrator1/1  "v"
  resting membrane potential/1 -> Add2/2, Add/2
  AHP or ADP/1 -> reset function/2(c)
  Add2/1 -> Product/1
  reset function/3(r) -> Integrator1/2, Integrator/2, output/1
  Gain1/1 -> f''/1
  Add3/1 -> Product/2
  Memory1/1 -> reset function/1(v)
  reset function/1(v1) -> Add/1, Add2/1, Add3/1
  reset function/2(u1) -> f''/2, f'/3
  Memory/1 -> reset function/4(u)
  Add/1 -> Gain1/1
  Integrator/1 -> Memory/1  "u"
  AP threshold potential/1 -> Add3/2
  Integrator1/1 -> v/1, Memory1/1  "v"
  f'/1 -> membrne capacitance/1
  Product/1 -> Gain2/1
  Gain2/1 -> f'/2
  postsynaptic current/1 -> f'/1

== system pattern_separation/granule cell 2/single exp EPSCs generator (recurrent synapse) ==
  event time : Inport
  decay time constant : Inport  Port=2
  conductance maximum : Inport  Port=3
  Add1 : Sum  Inputs=+-
  MATLAB Function : MATLAB Function  TreatAsAtomicUnit=on
  Multiply : Gain  Gain=-1
  Product : Product
  Product1 : Product  Inputs=*/
  Product2 : Product
  current reversal potential : Constant  Value=ve1  SampleTime=-1
  resting membrane potential : Constant  Value=vr1  SampleTime=-1
  postsynaptic current : Outport
  wires:
  decay time constant/1 -> Product1/2
  Product/1 -> postsynaptic current/1  "postsynaptic current"
  resting membrane potential/1 -> Add1/1
  current reversal potential/1 -> Add1/2
  conductance maximum/1 -> Product2/2
  Product2/1 -> Product/2  "conductance"
  Add1/1 -> Multiply/1
  Product1/1 -> MATLAB Function/1(inp)
  MATLAB Function/1(exponential) -> Product2/1
  event time/1 -> Product1/1
  Multiply/1 -> Product/1

== system pattern_separation/granule cell 2/single exp IPSCs generator (ihibitory synapse) ==
  event time : Inport
  decay time constant : Inport  Port=2
  conductance maximum : Inport  Port=3
  Add1 : Sum  Inputs=+-
  MATLAB Function : MATLAB Function  TreatAsAtomicUnit=on
  Multiply : Gain  Gain=-1
  Product : Product
  Product1 : Product  Inputs=*/
  Product2 : Product
  current reversal potential : Constant  Value=ve2  SampleTime=-1
  resting membrane potential : Constant  Value=vr2  SampleTime=-1
  postsynaptic current : Outport
  wires:
  decay time constant/1 -> Product1/2
  Product/1 -> postsynaptic current/1  "postsynaptic current"
  resting membrane potential/1 -> Add1/1
  current reversal potential/1 -> Add1/2
  conductance maximum/1 -> Product2/2
  Product2/1 -> Product/2  "conductance"
  Add1/1 -> Multiply/1
  Product1/1 -> MATLAB Function/1(inp)
  MATLAB Function/1(exponential) -> Product2/1
  event time/1 -> Product1/1
  Multiply/1 -> Product/1
